simulink model "WareHouseTaskRobotSimulationModel"  (R2024b)
settings: Solver=FixedStepAuto  StartTime=0.0  StopTime=250  FixedStep=0.1  RelTol=1e-3
PreLoadFcn:
  | load warehouseMaps.mat logicalMap
  | map = binaryOccupancyMap(logicalMap);
  | 
  | chargingStn = [5,5];
  | loadingStn = [52,15];
  | unloadingStn = [15,42];
  | 
  | angularVelFaultGain = 2;
StartFcn:
  | close all
StopFcn:
  | runIds = Simulink.sdi.getAllRunIDs;
  | lastRun = Simulink.sdi.getRun(runIds(end));
  | data = lastRun.getSignalsByName('state').Values.Data;
  | hold on;
  | plot(data(:,1), data(:,2),'LineWidth',2);
undefined symbols (not defined in the file): logicalMap
libraries: robotmobilelib x1
settings Model: Creator=marcob  LastModifiedBy=mbecker
settings OptimizationCC: BlockReduction=off  ConditionallyExecuteInputs=off
settings DebuggingCC: AlgebraicLoopMsg=error

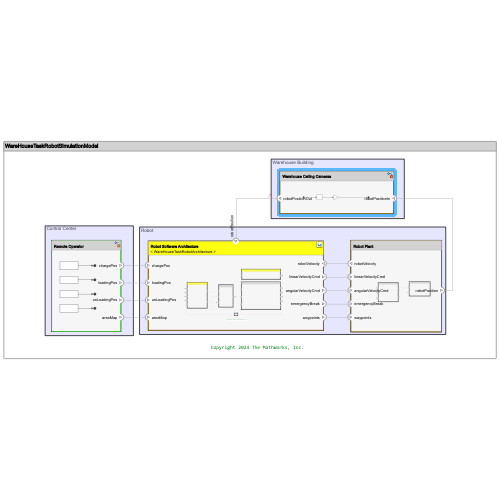
[thumbnail: Simulink's stored preview of the top-level diagram]
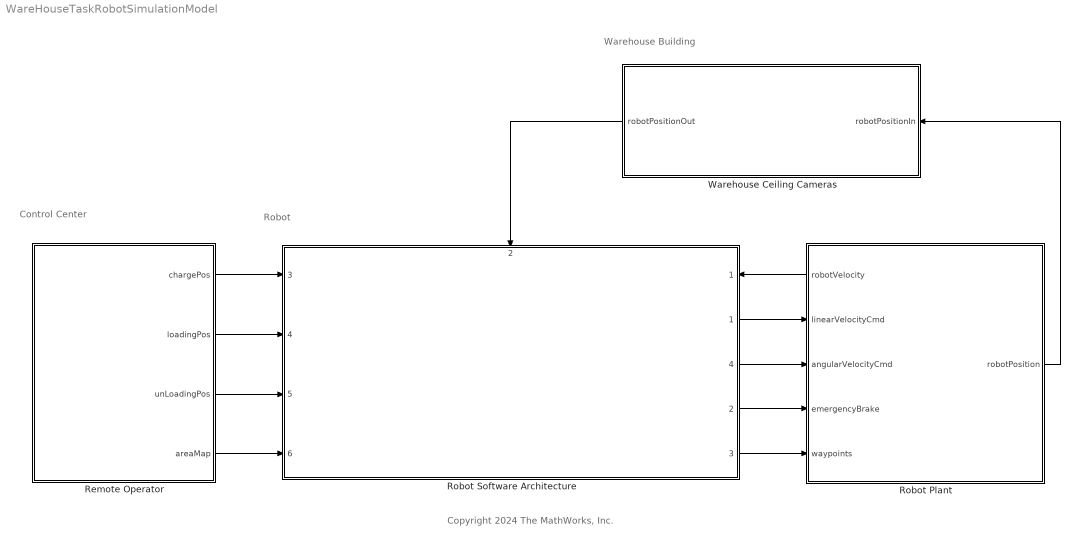
== system WareHouseTaskRobotSimulationModel ==
  note: Warehouse Building
  note: Robot
  note: Control Center
  note: Copyright 2024 The MathWorks, Inc.
  Remote Operator : Subsystem
      settings: PortSchema="{\"entries\":[{\"content\":{\"headerSize\":26,\"margin\":15,\"minimumSpacing\":25,\"sides\":[{\"content\":{},\"type\":\"ConnectorPlacement.EquallySpacedRectSide\",\"uuid\":\"fee8ae93-d3af-4af3-aba8-8bbb6c49b1e5\"},{\"content\":{\"connectorIds\":[\"Out1\",\"Out2\",\"Out3\",\"Out4\"],\"side\":\"RIGHT\"},\"type\":\"ConnectorPlacement.EquallySpacedRectSide\",\"uuid\":\"b0456245-7dcd-4816-a6fb-4f2f475968b2\"},{\"content\":{\"side\":\"TOP\"},\"type\":\"ConnectorPlacement.EquallySpacedRectSide\",\"uuid\":\"a975d676-5342-48fd-ad94-ed1438dae107\"}]},\"type\":\"ConnectorPlacement.EquallySpacedConnector\",\"uuid\":\"79662a43-5fa9-4b9c-9165-dcb3e1feed12\"}],\"packageUris\":[\"http://schema.mathworks.com/mf0/Connector/R2020b\"],\"version\":\"1.0\"}"
  Robot Plant : Subsystem
      settings: PortSchema="{\"entries\":[{\"content\":{\"headerSize\":26,\"margin\":15,\"minimumSpacing\":25,\"sides\":[{\"content\":{\"connectorIds\":[\"Out2\",\"In1\",\"In2\",\"In3\",\"In4\"]},\"type\":\"ConnectorPlacement.EquallySpacedRectSide\",\"uuid\":\"fee8ae93-d3af-4af3-aba8-8bbb6c49b1e5\"},{\"content\":{\"connectorIds\":[\"Out1\"],\"side\":\"RIGHT\"},\"type\":\"ConnectorPlacement.EquallySpacedRectSide\",\"uuid\":\"b0456245-7dcd-4816-a6fb-4f2f475968b2\"},{\"content\":{\"side\":\"TOP\"},\"type\":\"ConnectorPlacement.EquallySpacedRectSide\",\"uuid\":\"a975d676-5342-48fd-ad94-ed1438dae107\"}]},\"type\":\"ConnectorPlacement.EquallySpacedConnector\",\"uuid\":\"79662a43-5fa9-4b9c-9165-dcb3e1feed12\"}],\"packageUris\":[\"http://schema.mathworks.com/mf0/Connector/R2020b\"],\"version\":\"1.0\"}"
  Robot Software Architecture : Subsystem  ReferencedSubsystem=WareHouseTaskRobotArchitecture
      settings: PortSchema="{\"entries\":[{\"content\":{\"headerSize\":26,\"margin\":15,\"minimumSpacing\":25,\"sides\":[{\"content\":{\"connectorIds\":[\"In3\",\"In4\",\"In5\",\"In6\"]},\"type\":\"ConnectorPlacement.EquallySpacedRectSide\",\"uuid\":\"fee8ae93-d3af-4af3-aba8-8bbb6c49b1e5\"},{\"content\":{\"connectorIds\":[\"In1\",\"Out1\",\"Out4\",\"Out2\",\"Out3\"],\"side\":\"RIGHT\"},\"type\":\"ConnectorPlacement.EquallySpacedRectSide\",\"uuid\":\"b0456245-7dcd-4816-a6fb-4f2f475968b2\"},{\"content\":{\"connectorIds\":[\"In2\"],\"side\":\"TOP\"},\"type\":\"ConnectorPlacement.EquallySpacedRectSide\",\"uuid\":\"a975d676-5342-48fd-ad94-ed1438dae107\"}]},\"type\":\"ConnectorPlacement.EquallySpacedConnector\",\"uuid\":\"79662a43-5fa9-4b9c-9165-dcb3e1feed12\"}],\"packageUris\":[\"http://schema.mathworks.com/mf0/Connector/R2020b\"],\"version\":\"1.0\"}"
  Warehouse Ceiling Cameras : Subsystem
      settings: PortSchema="{\"entries\":[{\"content\":{\"headerSize\":26,\"margin\":15,\"minimumSpacing\":25,\"sides\":[{\"content\":{\"connectorIds\":[\"Out1\"]},\"type\":\"ConnectorPlacement.EquallySpacedRectSide\",\"uuid\":\"5ccff003-76f7-4779-807a-91871d9674a7\"},{\"content\":{\"connectorIds\":[\"In1\"],\"side\":\"RIGHT\"},\"type\":\"ConnectorPlacement.EquallySpacedRectSide\",\"uuid\":\"6cd9e982-3620-451d-98aa-950993e654a7\"},{\"content\":{\"side\":\"TOP\"},\"type\":\"ConnectorPlacement.EquallySpacedRectSide\",\"uuid\":\"2bbc8775-e2c4-4cb5-b84c-c760113c580e\"},{\"content\":{\"side\":\"BOTTOM\"},\"type\":\"ConnectorPlacement.EquallySpacedRectSide\",\"uuid\":\"829c0d19-c3bc-41ad-baca-5efe76fdbc9f\"}]},\"type\":\"ConnectorPlacement.EquallySpacedConnector\",\"uuid\":\"e16273e9-2f6a-4fc6-ae3c-1aa32184264a\"}],\"packageUris\":[\"http://schema.mathworks.com/mf0/Connector/R2020b\"],\"version\":\"1.0\"}"
  wires:
  Robot Software Architecture/1 -> Robot Plant/1(linearVelocityCmd)
  Robot Software Architecture/3 -> Robot Plant/4(waypoints)
  Robot Plant/2(robotVelocity) -> Robot Software Architecture/1
  Remote Operator/4(areaMap) -> Robot Software Architecture/6
  Remote Operator/1(chargePos) -> Robot Software Architecture/3
  Remote Operator/2(loadingPos) -> Robot Software Architecture/4
  Remote Operator/3(unLoadingPos) -> Robot Software Architecture/5
  Robot Software Architecture/4 -> Robot Plant/2(angularVelocityCmd)
  Robot Software Architecture/2 -> Robot Plant/3(emergencyBrake)
  Robot Plant/1(robotPosition) -> Warehouse Ceiling Cameras/1(robotPositionIn)
  Warehouse Ceiling Cameras/1(robotPositionOut) -> Robot Software Architecture/2

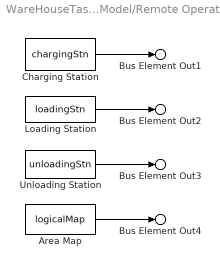
== system WareHouseTaskRobotSimulationModel/Remote Operator ==
  "Area Map " : Constant  Value=logicalMap  SampleTime=1
  "Charging Station " : Constant  Value=chargingStn  SampleTime=1
  Loading Station : Constant  Value=loadingStn
  Unloading Station : Constant  Value=unloadingStn  SampleTime=1
  Bus Element Out1 : Outport  PortName=chargePos
  Bus Element Out2 : Outport  Port=2  PortName=loadingPos
  Bus Element Out3 : Outport  Port=3  PortName=unLoadingPos
  Bus Element Out4 : Outport  Port=4  PortName=areaMap
  wires:
  "Charging Station "/1 -> Bus Element Out1/1
  Loading Station/1 -> Bus Element Out2/1
  Unloading Station/1 -> Bus Element Out3/1
  "Area Map "/1 -> Bus Element Out4/1

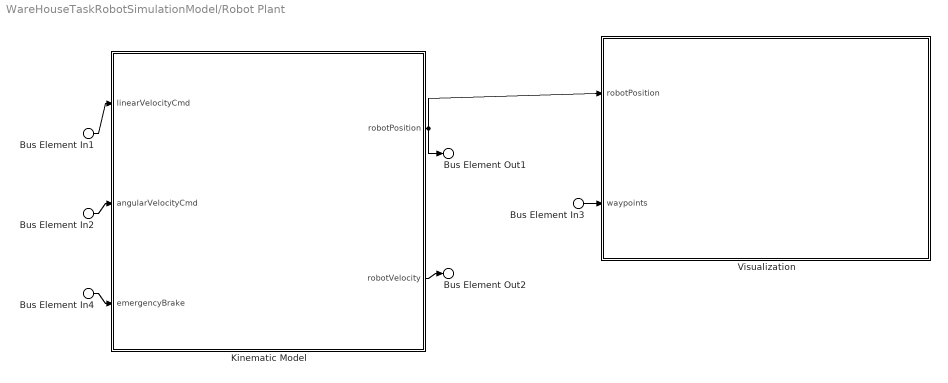
== system WareHouseTaskRobotSimulationModel/Robot Plant ==
  Bus Element In1 : Inport  PortName=linearVelocityCmd
  Bus Element In2 : Inport  Port=2  PortName=angularVelocityCmd
  Bus Element In4 : Inport  Port=3  PortName=emergencyBrake
  Bus Element In3 : Inport  Port=4  PortName=waypoints
  Kinematic Model : Subsystem
      settings: PortSchema="{\"entries\":[{\"content\":{\"headerSize\":26,\"margin\":15,\"minimumSpacing\":25,\"sides\":[{\"content\":{\"connectorIds\":[\"In1\",\"In2\",\"In3\"]},\"type\":\"ConnectorPlacement.EquallySpacedRectSide\",\"uuid\":\"fee8ae93-d3af-4af3-aba8-8bbb6c49b1e5\"},{\"content\":{\"connectorIds\":[\"Out1\",\"Out2\"],\"side\":\"RIGHT\"},\"type\":\"ConnectorPlacement.EquallySpacedRectSide\",\"uuid\":\"b0456245-7dcd-4816-a6fb-4f2f475968b2\"},{\"content\":{\"side\":\"TOP\"},\"type\":\"ConnectorPlacement.EquallySpacedRectSide\",\"uuid\":\"a975d676-5342-48fd-ad94-ed1438dae107\"}]},\"type\":\"ConnectorPlacement.EquallySpacedConnector\",\"uuid\":\"79662a43-5fa9-4b9c-9165-dcb3e1feed12\"}],\"packageUris\":[\"http://schema.mathworks.com/mf0/Connector/R2020b\"],\"version\":\"1.0\"}"
  Visualization : Subsystem
      settings: PortSchema="{\"entries\":[{\"content\":{\"headerSize\":26,\"margin\":15,\"minimumSpacing\":25,\"sides\":[{\"content\":{\"connectorIds\":[\"In1\",\"In2\"]},\"type\":\"ConnectorPlacement.EquallySpacedRectSide\",\"uuid\":\"fee8ae93-d3af-4af3-aba8-8bbb6c49b1e5\"},{\"content\":{\"side\":\"RIGHT\"},\"type\":\"ConnectorPlacement.EquallySpacedRectSide\",\"uuid\":\"b0456245-7dcd-4816-a6fb-4f2f475968b2\"},{\"content\":{\"side\":\"TOP\"},\"type\":\"ConnectorPlacement.EquallySpacedRectSide\",\"uuid\":\"a975d676-5342-48fd-ad94-ed1438dae107\"}]},\"type\":\"ConnectorPlacement.EquallySpacedConnector\",\"uuid\":\"79662a43-5fa9-4b9c-9165-dcb3e1feed12\"}],\"packageUris\":[\"http://schema.mathworks.com/mf0/Connector/R2020b\"],\"version\":\"1.0\"}"
  Bus Element Out1 : Outport  PortName=robotPosition
  Bus Element Out2 : Outport  Port=2  PortName=robotVelocity
  wires:
  Bus Element In2/1 -> Kinematic Model/2(angularVelocityCmd)
  Bus Element In1/1 -> Kinematic Model/1(linearVelocityCmd)
  Kinematic Model/1(robotPosition) -> Bus Element Out1/1, Visualization/1(robotPosition)
  Kinematic Model/2(robotVelocity) -> Bus Element Out2/1
  Bus Element In3/1 -> Visualization/2(waypoints)
  Bus Element In4/1 -> Kinematic Model/3(emergencyBrake)

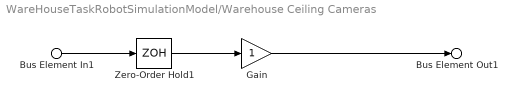
== system WareHouseTaskRobotSimulationModel/Warehouse Ceiling Cameras ==
  Bus Element In1 : Inport  PortName=robotPositionIn
  Gain : Gain
  Zero-Order Hold1 : ZeroOrderHold  SampleTime=-1
  Bus Element Out1 : Outport  PortName=robotPositionOut
  wires:
  Bus Element In1/1 -> Zero-Order Hold1/1
  Gain/1 -> Bus Element Out1/1
  Zero-Order Hold1/1 -> Gain/1

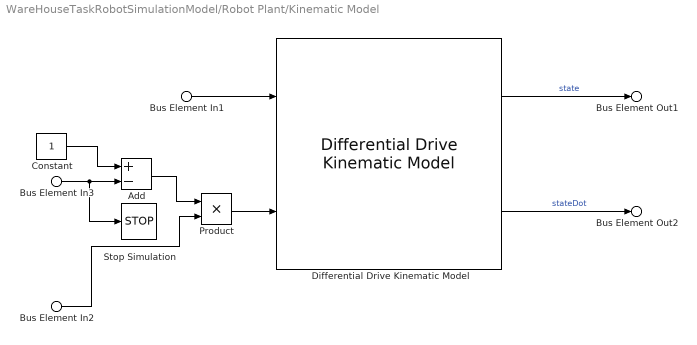
== system WareHouseTaskRobotSimulationModel/Robot Plant/Kinematic Model ==
  Bus Element In1 : Inport  PortName=linearVelocityCmd
  Bus Element In2 : Inport  Port=2  PortName=angularVelocityCmd
  Bus Element In3 : Inport  Port=3  PortName=emergencyBrake
  Add : Sum  Inputs=+-
  Constant : Constant
  "Differential Drive Kinematic Model " : robotmobilelib/Differential Drive Kinematic Model  VehicleInputs=Vehicle Speed & Heading Angular Velocity  WheelRadius=0.1  WheelSpeedRange=[-inf inf]  TrackWidth=0.3  InitialState=[chargingStn,0]'  SimulateUsing=Code generation
  Product : Product
  Stop Simulation : Stop
  Bus Element Out1 : Outport  PortName=robotPosition
  Bus Element Out2 : Outport  Port=2  PortName=robotVelocity
  wires:
  Bus Element In1/1 -> "Differential Drive Kinematic Model "/1
  "Differential Drive Kinematic Model "/1 -> Bus Element Out1/1  "state"
  "Differential Drive Kinematic Model "/2 -> Bus Element Out2/1  "stateDot"
  Product/1 -> "Differential Drive Kinematic Model "/2
  Constant/1 -> Add/1
  Bus Element In3/1 -> Add/2, Stop Simulation/1
  Add/1 -> Product/1
  Bus Element In2/1 -> Product/2

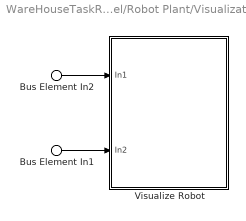
== system WareHouseTaskRobotSimulationModel/Robot Plant/Visualization ==
  Bus Element In2 : Inport  PortName=robotPosition
  Bus Element In1 : Inport  Port=2  PortName=waypoints
  Visualize Robot : Subsystem  mask{MeshSelectionIdx=Ground vehicle, PresetViews=Entire Map, ShowViz=on, ShowPaths=on, MapXMin=0, MapXMax=60, MapYMin=0, MapYMax=60, XLimits=[0 size(logicalMap, 1)], YLimits=[0 size(logicalMap, 2)], LocalXLimits=[-10 10], LocalYLimits=[-10 10], ChargingLocation=chargingStn, SortingStation=loadingStn, UnloadingStation=unloadingStn, VisualizationSampleRate=5}
      mask prompts: MeshSelectionIdx "Robot mesh"; PresetViews "Preset Views"; ShowViz "Update visualization:"; ShowPaths "Show planned paths:"; MapXMin "Map xmin:"; MapXMax "Map xmax:"; MapYMin "Map ymin:"; MapYMax "Map ymax:"; XLimits "Map x-limits:"; YLimits "Map y-limits:"; LocalXLimits "Local view x-limits"; LocalYLimits "Local view y-limits"; ChargingLocation "Start locations:"; SortingStation "Dock locations:"; UnloadingStation "Shelf locations:"; VisualizationSampleRate "Sample time:"
      mask init:
      | % Create the list of key locations
      | startLocationMatrix = evalin('base', get_param(gcb, 'ChargingLocation'));
      | shelfLocationMatrix = evalin('base', get_param(gcb, 'UnloadingStation'));
      | dockLocationMatrix = evalin('base', get_param(gcb, 'SortingStation'));
      | 
      | % Create popup list from matrices
      | dockLocationNameCell = cell(size(dockLocationMatrix,1),1);
      | shelfLocationNameCell = cell(size(shelfLocationMatrix,1),1);
      | startLocationNameCell = cell(size(startLocationMatrix,1),1);
      | for i = 1:size(startLocationMatrix,1)
      |     startLocationNameCell{i} = ['Charging Station ' num2str(i)];
      | end
      | for j = 1:size(shelfLocationMatrix,1)
      |     shelfLocationNameCell{j} = ['Unloading Station ' num2str(j)];
      | end
      | for k = 1:size(dockLocationMatrix,1)
      |     dockLocationNameCell{k} = ['Sorting Station ' num2str(k)];
      | end
      | 
      | % Update the parameter list
      | m = Simulink.Mask.get(gcb);
      | viewPopupParam = m.getParameter('PresetViews');
      | viewPopupParam.TypeOptions = [...
      |     {'Entire Map'}; ...
      |     dockLocationNameCell; ...
      |     shelfLocationNameCell; ...
      |     startLocationNameCell ... 
      |     ];
      mask TypeOptions MeshSelectionIdx: Ground vehicle | Forklift
      mask TypeOptions PresetViews: Entire Map | Sorting Station 1 | Unloading Station 1 | Charging Station 1
      mask Callback PresetViews:
      | % Get key numeric data
      | startLocationMatrix = evalin('base', get_param(gcb, 'ChargingLocation'));
      | dockLocationMatrix = evalin('base', get_param(gcb, 'SortingStation'));
      | shelfLocationMatrix = evalin('base', get_param(gcb, 'UnloadingStation'));
      | mapXLim = evalin('base', get_param(gcb, 'XLimits'));
      | mapYLim = evalin('base', get_param(gcb, 'YLimits'));
      | viewXLim = evalin('base', get_param(gcb, 'LocalXLimits'));
      | viewYLim = evalin('base', get_param(gcb, 'LocalYLimits'));
      | 
      | % Get selected value
      | viewSelection = get_param(gcb, 'PresetViews');
      | 
      | %Take action based on view
      | if strcmp(viewSelection, 'Custom')
      |     % Do nothing
      | else
      |     if strcmp(viewSelection(1:5), 'Charg')
      |         % Start location
      |         startIndex = str2double(viewSelection(end));
      |         localPts = startLocationMatrix(startIndex, :);
      |         viewLimits = [localPts(1)+viewXLim(1) localPts(1)+viewXLim(2) ...
      |             localPts(2)+viewYLim(1) localPts(2)+viewYLim(2)];
      | 
      |     elseif strcmp(viewSelection(1:5), 'Sorti')
      |         % Dock (Loading) location
      |         dockIndex = str2double(viewSelection(end));
      |         localPts = dockLocationMatrix(dockIndex, :);
      |         viewLimits = [localPts(1)+viewXLim(1) localPts(1)+viewXLim(2) ...
      |             localPts(2)+viewYLim(1) localPts(2)+viewYLim(2)];
      | 
      |     elseif strcmp(viewSelection(1:5), 'Unloa')
      |         % Shelf (Unloading) location
      |         shelfIndex = str2double(viewSelection(end));
      |         localPts = shelfLocationMatrix(shelfIndex, :);
      |         viewLimits = [localPts(1)+viewXLim(1) localPts(1)+viewXLim(2) ...
      |             localPts(2)+viewYLim(1) localPts(2)+viewYLim(2)];
      | 
      |     else
      |         % Show the whole map
      |         viewLimits = [mapXLim(1) mapXLim(2) mapYLim(1) mapYLim(2)];
      |     end
      | 
      |     % Set the map parameters
      |     set_param(gcb, 'MapXMin', num2str(viewLimits(1)));
      |     set_param(gcb, 'MapXMax', num2str(viewLimits(2)));
      |     set_param(gcb, 'MapYMin', num2str(viewLimits(3)));
      |     set_param(gcb, 'MapYMax', num2str(viewLimits(4)));
      | end
      mask Callback MapXMin:
      | currentMax = str2num(get_param(gcb, 'MapXMax'));
      | newMin = str2num(get_param(gcb, 'MapXMin'));
      | if newMin > currentMax
      |     set_param(gcb, 'MapXMax', num2str(newMin+1));
      | end
      mask Callback MapXMax:
      | currentMin = str2num(get_param(gcb, 'MapXMin'));
      | newMax = str2num(get_param(gcb, 'MapXMax'));
      | if newMax < currentMin
      |     set_param(gcb, 'MapXMin', num2str(newMax-1));
      | end
      mask Callback MapYMin:
      | currentMax = str2num(get_param(gcb, 'MapYMax'));
      | newMin = str2num(get_param(gcb, 'MapYMin'));
      | if newMin > currentMax
      |     set_param(gcb, 'MapYMax', num2str(newMin+1));
      | end
      mask Callback MapYMax:
      | currentMin = str2num(get_param(gcb, 'MapYMin'));
      | newMax = str2num(get_param(gcb, 'MapYMax'));
      | if newMax < currentMin
      |     set_param(gcb, 'MapYMin', num2str(newMax-1));
      | end
      mask DialogControl DescGroupVar Prompt: Visualization example helper
      mask DialogControl DescTextVar Prompt: This subsystem plots the robots and environement and allows users to change the views.
      mask DialogControl ViewLimits Prompt: View limits
      mask DialogControl ViewConfigurationGroup Prompt: View configuration:
      mask DialogControl ViewParamSourcesGroup Prompt: View parameter sources
      mask Display: disp('Visualization Helper')
  wires:
  Bus Element In2/1 -> Visualize Robot/1(In1)
  Bus Element In1/1 -> Visualize Robot/2(In2)

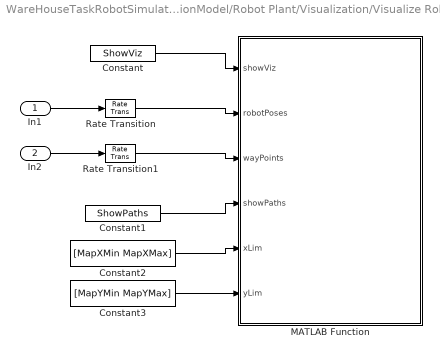
== system WareHouseTaskRobotSimulationModel/Robot Plant/Visualization/Visualize Robot ==
  In1 : Inport
  In2 : Inport  Port=2
  Constant : Constant  Value=ShowViz
  Constant1 : Constant  Value=ShowPaths
  Constant2 : Constant  Value=[MapXMin MapXMax]
  Constant3 : Constant  Value=[MapYMin MapYMax]
  MATLAB Function : MATLAB Function  TreatAsAtomicUnit=on
  Rate Transition : RateTransition
  Rate Transition1 : RateTransition
  wires:
  In2/1 -> Rate Transition1/1
  In1/1 -> Rate Transition/1
  Rate Transition/1 -> MATLAB Function/2(robotPoses)
  Rate Transition1/1 -> MATLAB Function/3(wayPoints)
  Constant/1 -> MATLAB Function/1(showViz)
  Constant1/1 -> MATLAB Function/4(showPaths)
  Constant2/1 -> MATLAB Function/5(xLim)
  Constant3/1 -> MATLAB Function/6(yLim)

== matlab function WareHouseTaskRobotSimulationModel/Robot Plant/Visualization/Visualize Robot/MATLAB Function ==
  settings: updateMethod=DISCRETE  sampleTime=VisualizationSampleRate
  data: showViz input; robotPoses input; wayPoints input; logicalMap parameter; ChargingLocation parameter; UnloadingStation parameter; SortingStation parameter; showPaths input; xLim input; yLim input; MeshSelectionIdx parameter
function simulationVisualization(showViz, robotPoses, wayPoints, logicalMap, ChargingLocation, UnloadingStation, SortingStation, showPaths, xLim, yLim, MeshSelectionIdx)
%#codegen

%% Setup

coder.extrinsic('exampleHelperVisualizeExecuteRobots');
persistent f
if isempty(f) && showViz
    f = figure('units','normalized','outerposition',[0 0 0.75 0.75]);
    title('Mobile Robot Motion');
    set(f, 'Visible', 'on');
end

% Robot mesh options are cells of the unloaded and loaded robot mesh and
% the translation between the visualized origin and the desired origin
meshOptions = {...
    {'groundvehicle.stl', [.314 0 .155], 'groundvehiclewithload.stl', [.312 0 .156]}, ...
    {'forkliftExecuteRobotTasks.stl', [.3569 0 .297], 'forkliftwithload.stl', [.3813 0 .2893]}, ...
    };
    

if showViz && ~isempty(f)
    exampleHelperVisualizeExecuteRobots(f, robotPoses, wayPoints, logicalMap, ChargingLocation, UnloadingStation, SortingStation, showPaths, xLim, yLim, meshOptions{MeshSelectionIdx});
end
end
